simulink model "PIPTB_simulation"  (R2020b)
settings: Solver=FixedStepAuto  StartTime=0.0  StopTime=1.5  FixedStep=0.001  RelTol=1e-3
values from neighbouring files (symbols this model uses):
  C = eye(4,4)    [Derive_PIPTB_Model.m]
  D = zeros(4,1)    [Derive_PIPTB_Model.m]
  K = [-46.14 0 -7.4 -1.998]    [LQR_calculation.m]
  x0 = [0/180*pi; 0; 0; 0]    [LQR_calculation.m]
undefined symbols (not defined in the file or in its folder): AA, BB
libraries: simulink x2
settings Model: Creator=cxiao3  LastModifiedBy=cxiao3
settings SFSimCC: CustomCodeUndefinedFunction=UseInterfaceOnly

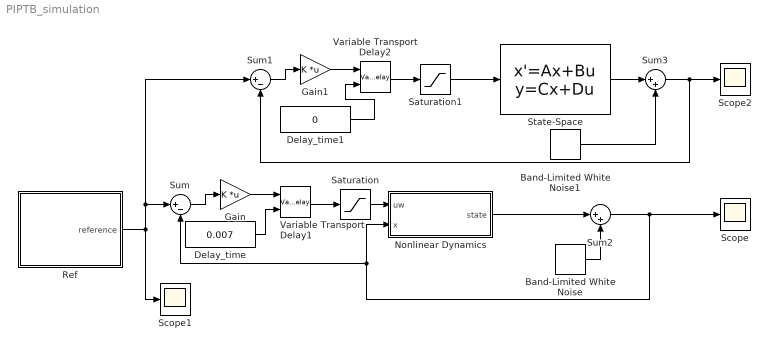
== system PIPTB_simulation ==
  Band-Limited White Noise : simulink/Sources/Band-Limited White Noise  Cov=[1E-8]  Ts=0.001  seed=[23341]
  Band-Limited White Noise1 : simulink/Sources/Band-Limited White Noise  Cov=[1E-8]  Ts=0.001  seed=[23341]
  Delay_time : Constant  Value=0.007
  Delay_time1 : Constant  Value=0
  Gain : Gain  Gain=K  Multiplication=Matrix(K*u)
  Gain1 : Gain  Gain=K  Multiplication=Matrix(K*u)
  Nonlinear Dynamics : Subsystem
  Ref : Subsystem
  Saturation : Saturate  UpperLimit=5  LowerLimit=-5
  Saturation1 : Saturate  UpperLimit=5  LowerLimit=-5
  Scope : Scope
  Scope1 : Scope
  Scope2 : Scope
  State-Space : StateSpace  A=AA  B=BB  C=C  D=D  InitialCondition=0
  Sum : Sum  Inputs=|+-
  Sum1 : Sum  Inputs=|+-
  Sum2 : Sum  Inputs=|++
  Sum3 : Sum  Inputs=|++
  Variable Transport Delay1 : VariableTransportDelay  MaximumDelay=10  ZeroDelay=on
  Variable Transport Delay2 : VariableTransportDelay  MaximumDelay=10  ZeroDelay=on
  wires:
  Nonlinear Dynamics/1(state) -> Sum2/1
  Band-Limited White Noise/1 -> Sum2/2
  Sum2/1 -> Sum/2, Nonlinear Dynamics/2(x), Scope/1
  Variable Transport Delay1/1 -> Saturation/1
  Delay_time/1 -> Variable Transport Delay1/2
  Gain/1 -> Variable Transport Delay1/1
  Saturation/1 -> Nonlinear Dynamics/1(uw)
  Sum/1 -> Gain/1
  Sum1/1 -> Gain1/1
  Delay_time1/1 -> Variable Transport Delay2/2
  Gain1/1 -> Variable Transport Delay2/1
  Variable Transport Delay2/1 -> Saturation1/1
  Ref/1(reference) -> Scope1/1, Sum1/1, Sum/1
  Saturation1/1 -> State-Space/1
  State-Space/1 -> Sum3/1
  Sum3/1 -> Scope2/1, Sum1/2
  Band-Limited White Noise1/1 -> Sum3/2

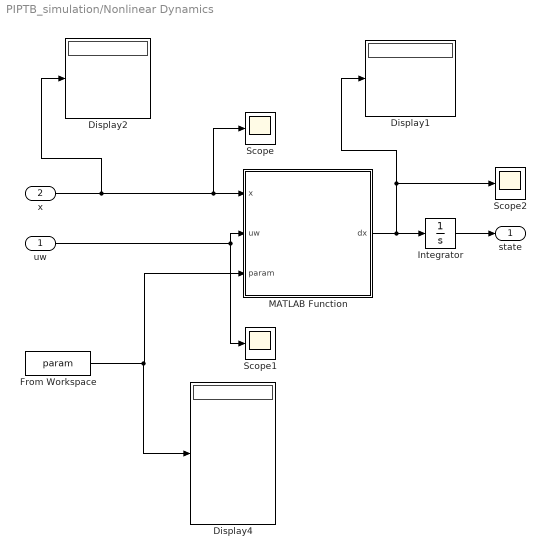
== system PIPTB_simulation/Nonlinear Dynamics ==
  uw : Inport
  x : Inport  Port=2
  Display1 : Display
  Display2 : Display
  Display4 : Display
  From Workspace : FromWorkspace  VariableName=param
  Integrator : Integrator  InitialCondition=x0
  MATLAB Function : MATLAB Function  TreatAsAtomicUnit=on
  Scope : Scope
  Scope1 : Scope
  Scope2 : Scope
  state : Outport  VectorParamsAs1DForOutWhenUnconnected=off
  wires:
  MATLAB Function/1(dx) -> Display1/1, Scope2/1, Integrator/1
  Integrator/1 -> state/1
  x/1 -> Display2/1, Scope/1, MATLAB Function/1(x)
  From Workspace/1 -> Display4/1, MATLAB Function/3(param)
  uw/1 -> MATLAB Function/2(uw), Scope1/1

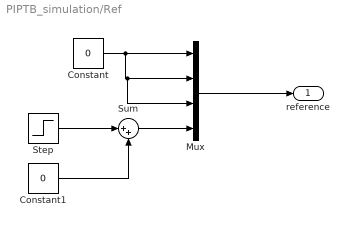
== system PIPTB_simulation/Ref ==
  Constant : Constant  Value=0
  Constant1 : Constant  Value=0
  Mux : Mux
  Step : Step  Time=0.278  After=4  SampleTime=0
  Sum : Sum  Inputs=|++
  reference : Outport  VectorParamsAs1DForOutWhenUnconnected=off
  wires:
  Mux/1 -> reference/1
  Constant/1 -> Mux/3, Mux/2, Mux/1
  Step/1 -> Sum/1
  Sum/1 -> Mux/4
  Constant1/1 -> Sum/2

== matlab function PIPTB_simulation/Nonlinear Dynamics/MATLAB Function ==
  data: x input; dx output; uw input; param input
function dx = PIPTBDynamics(x,uw,param)
mK = param(1);
IK = param(2);
rK = param(3);
mA = param(4);
IA = param(5);
lAC = param(6);
mL = param(7);
g =9.8;
theta = x(1,:);  
phi = x(2,:);
dtheta = x(3,:);
dphi = x(4,:);
q = [theta;phi];
dq = [dtheta;dphi];

[ddtheta,ddphi] = autoGen_PIPTBDynamics(q,dq,uw,mK,IK,rK,mA,IA,lAC,mL,g);

dx = [dtheta;dphi;ddtheta;ddphi];

end
